simulink model "ntm"  (R2020a)
settings: Solver=VariableStepAuto  StartTime=0.0  StopTime=300  RelTol=1e-3
undefined symbols (not defined in the file or in its folder): National_Instruments, PCI
libraries: sldrtlib x5, simulink x2
settings Model: Creator=m_olivei  LastModifiedBy=m_olivei

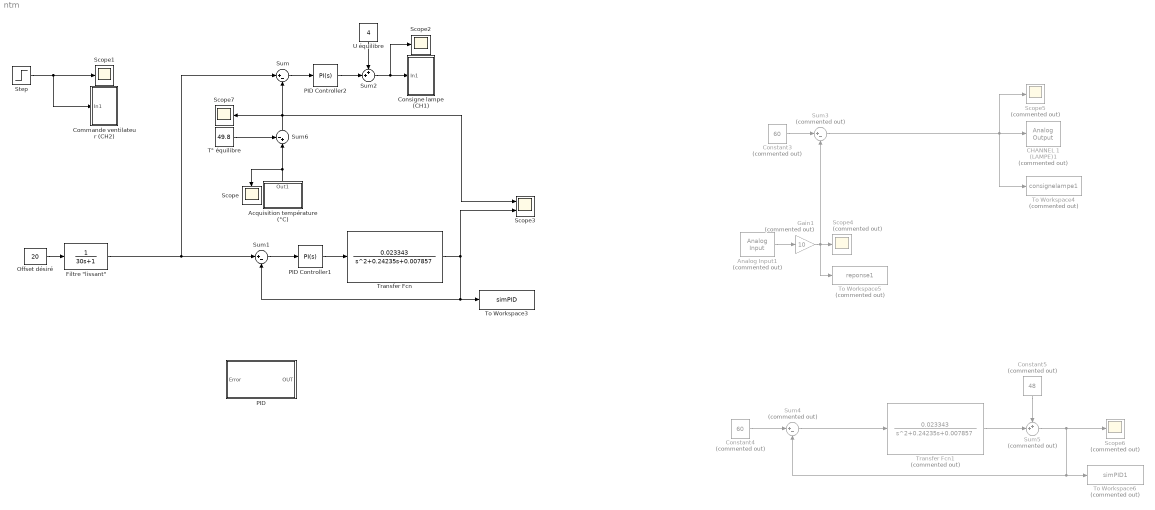
== system ntm ==
  Acquisition température (°C) : Subsystem
  Analog Input1 : sldrtlib/Analog Input  Commented=on  SampleTime=0.1  MaxMissedTicks=10  ShowMissedTicks=off  YieldWhenWaiting=off  DrvName=National_Instruments/PCI-6024E  DrvAddress=4294967295  DrvOptions=[0 0 0 0 0 0]  Channels=1  RangeMode=1  VoltRange=1  DataType=1
      settings: AttributesFormatString=National Instruments\nPCI-6024E [auto]
  CHANNEL 1 (LAMPE)1 : sldrtlib/Analog Output  Commented=on  SampleTime=0.1  MaxMissedTicks=10  ShowMissedTicks=off  YieldWhenWaiting=off  DrvName=National_Instruments/PCI-6024E  DrvAddress=4294967295  DrvOptions=[0 0 0 0 0 0]  Channels=1  RangeMode=1  VoltRange=1  InitialValue=[]  FinalValue=4
      settings: AttributesFormatString=National Instruments\nPCI-6024E [auto]
  Commande ventilateur (CH2) : Subsystem
  Consigne lampe (CH1) : Subsystem
  Constant3 : Constant  Commented=on  Value=60
  Constant4 : Constant  Commented=on  Value=60
  Constant5 : Constant  Commented=on  Value=48
  "Filtre \"lissant\"" : TransferFcn  Denominator=[30 1]
  Gain1 : Gain  Commented=on  Gain=10
  Offset désiré : Constant  Value=20
  PID : Subsystem
  PID Controller1 : simulink/Continuous/PID Controller  Controller=PI  Form=Parallel  TimeDomain=Continuous-time  UseExternalTs=off  SampleTime=-1  IntegratorMethod=Forward Euler  FilterMethod=Forward Euler  ControllerParametersSource=internal  P=0.134524809636123  I=0.0118548404136242  D=0  UseFilter=on  N=100  TunerSelectOption=Transfer Function Based (PID Tuner App)  InitialConditionSource=internal  InitialConditionForIntegrator=0  InitialConditionForFilter=0  DifferentiatorICPrevScaledInput=0  ExternalReset=none  TrackingMode=off  Kt=1  LimitOutput=on  UpperSaturationLimit=10  LowerSaturationLimit=0  LinearizeAsGain=on  AntiWindupMode=back-calculation  Kb=0.0118548404136242  POutMin=[]  POutMax=[]  IOutMin=[]  IOutMax=[]  DOutMin=[]  DOutMax=[]  NOutMin=[]  NOutMax=[]  SumOutMin=[]  SumOutMax=[]  SaturationOutMin=[]  SaturationOutMax=[]  PParamMin=[]  PParamMax=[]  IParamMin=[]  IParamMax=[]  DParamMin=[]  DParamMax=[]  NParamMin=[]  NParamMax=[]  KbParamMin=[]  KbParamMax=[]  KtParamMin=[]  KtParamMax=[]  KbOutMin=[]  KbOutMax=[]  KtOutMin=[]  KtOutMax=[]  IntegratorOutMin=[]  IntegratorOutMax=[]  FilterOutMin=[]  FilterOutMax=[]  SumI1OutMin=[]  SumI1OutMax=[]  SumI2OutMin=[]  SumI2OutMax=[]  SumI3OutMin=[]  SumI3OutMax=[]  SumI4OutMin=[]  SumI4OutMax=[]  SumDOutMin=[]  SumDOutMax=[]  DifferentiatorOutMin=[]  DifferentiatorOutMax=[]  FilterDiffOutCoefMin=[]  FilterDiffOutCoefMax=[]  ReciprocalOutMin=[]  ReciprocalOutMax=[]  SumDenOutMin=[]  SumDenOutMax=[]  SumNumOutMin=[]  SumNumOutMax=[]  DivideOutMin=[]  DivideOutMax=[]  UdiffTsProdOutMin=[]  UdiffTsProdOutMax=[]  NTsProdOutMin=[]  NTsProdOutMax=[]  UintegralTsProdOutMin=[]  UintegralTsProdOutMax=[]  UngainTsProdOutMin=[]  UngainTsProdOutMax=[]  IntegratorContinuousStateAttributes=''  IntegratorStateMustResolveToSignalObject=off  IntegratorRTWStateStorageClass=Auto  FilterContinuousStateAttributes=''  FilterStateMustResolveToSignalObject=off  FilterRTWStateStorageClass=Auto  ParallelPVariant=InternalParameters  IdealPVariant=Disabled  IVariant=InternalParameters  DVariant=Disabled  IntegratorVariant=Continuous  SatVariant=Enabled  AWVariant=BackCalculation  PCopyVariant=Disabled  TRVariant=Disabled  FdbkBlocksVariant=Forward  IdealPFdbkVariant=Disabled  SatFdbkVariant=Disabled  DerivativeFilterVariant=Disabled  NVariant=Disabled  NCopyVariant=Disabled_SignalSpec  FilterICVariant=Disabled  IntegratorICVariant=InternalICs  ExternalResetVariant=Disabled  TRSumVariant=Passthrough  SumFdbkVariant=Disabled  SumVariant=Sum_PI  TsampFilterVariant=InternalTs  TsampNgainVariant=Passthrough  TsampIntegralVariant=Passthrough
  PID Controller2 : simulink/Continuous/PID Controller  Controller=PI  Form=Parallel  TimeDomain=Continuous-time  UseExternalTs=off  SampleTime=-1  IntegratorMethod=Forward Euler  FilterMethod=Forward Euler  ControllerParametersSource=internal  P=0.134524809636123  I=0.0118548404136242  D=0  UseFilter=on  N=100  TunerSelectOption=Transfer Function Based (PID Tuner App)  InitialConditionSource=internal  InitialConditionForIntegrator=0  InitialConditionForFilter=0  DifferentiatorICPrevScaledInput=0  ExternalReset=none  TrackingMode=off  Kt=1  LimitOutput=on  UpperSaturationLimit=6  LowerSaturationLimit=0  LinearizeAsGain=on  AntiWindupMode=back-calculation  Kb=0.0118548404136242  POutMin=[]  POutMax=[]  IOutMin=[]  IOutMax=[]  DOutMin=[]  DOutMax=[]  NOutMin=[]  NOutMax=[]  SumOutMin=[]  SumOutMax=[]  SaturationOutMin=[]  SaturationOutMax=[]  PParamMin=[]  PParamMax=[]  IParamMin=[]  IParamMax=[]  DParamMin=[]  DParamMax=[]  NParamMin=[]  NParamMax=[]  KbParamMin=[]  KbParamMax=[]  KtParamMin=[]  KtParamMax=[]  KbOutMin=[]  KbOutMax=[]  KtOutMin=[]  KtOutMax=[]  IntegratorOutMin=[]  IntegratorOutMax=[]  FilterOutMin=[]  FilterOutMax=[]  SumI1OutMin=[]  SumI1OutMax=[]  SumI2OutMin=[]  SumI2OutMax=[]  SumI3OutMin=[]  SumI3OutMax=[]  SumI4OutMin=[]  SumI4OutMax=[]  SumDOutMin=[]  SumDOutMax=[]  DifferentiatorOutMin=[]  DifferentiatorOutMax=[]  FilterDiffOutCoefMin=[]  FilterDiffOutCoefMax=[]  ReciprocalOutMin=[]  ReciprocalOutMax=[]  SumDenOutMin=[]  SumDenOutMax=[]  SumNumOutMin=[]  SumNumOutMax=[]  DivideOutMin=[]  DivideOutMax=[]  UdiffTsProdOutMin=[]  UdiffTsProdOutMax=[]  NTsProdOutMin=[]  NTsProdOutMax=[]  UintegralTsProdOutMin=[]  UintegralTsProdOutMax=[]  UngainTsProdOutMin=[]  UngainTsProdOutMax=[]  IntegratorContinuousStateAttributes=''  IntegratorStateMustResolveToSignalObject=off  IntegratorRTWStateStorageClass=Auto  FilterContinuousStateAttributes=''  FilterStateMustResolveToSignalObject=off  FilterRTWStateStorageClass=Auto  ParallelPVariant=InternalParameters  IdealPVariant=Disabled  IVariant=InternalParameters  DVariant=Disabled  IntegratorVariant=Continuous  SatVariant=Enabled  AWVariant=BackCalculation  PCopyVariant=Disabled  TRVariant=Disabled  FdbkBlocksVariant=Forward  IdealPFdbkVariant=Disabled  SatFdbkVariant=Disabled  DerivativeFilterVariant=Disabled  NVariant=Disabled  NCopyVariant=Disabled_SignalSpec  FilterICVariant=Disabled  IntegratorICVariant=InternalICs  ExternalResetVariant=Disabled  TRSumVariant=Passthrough  SumFdbkVariant=Disabled  SumVariant=Sum_PI  TsampFilterVariant=InternalTs  TsampNgainVariant=Passthrough  TsampIntegralVariant=Passthrough
  Scope{,1..2,7} (4 alike) : Scope
  Scope3 : Scope  NumInputPorts=2
  Scope4 : Scope  Commented=on
  Scope5 : Scope  Commented=on
  Scope6 : Scope  Commented=on
  Step : Step  SampleTime=0
  Sum : Sum  Inputs=|+-
  Sum1 : Sum  Inputs=|+-
  Sum2 : Sum  Inputs=++|
  Sum3 : Sum  Commented=on  Inputs=|+-
  Sum4 : Sum  Commented=on  Inputs=|+-
  Sum5 : Sum  Commented=on  Inputs=++|
  Sum6 : Sum  Inputs=-+|
  To Workspace3 : ToWorkspace  VariableName=simPID  SaveFormat=Timeseries  SampleTime=-1
  To Workspace4 : ToWorkspace  Commented=on  VariableName=consignelampe1  SaveFormat=Timeseries  SampleTime=-1
  To Workspace5 : ToWorkspace  Commented=on  VariableName=reponse1  SaveFormat=Timeseries  SampleTime=-1
  To Workspace6 : ToWorkspace  Commented=on  VariableName=simPID1  SaveFormat=Timeseries  SampleTime=-1
  Transfer Fcn : TransferFcn  Numerator=[0.023343]  Denominator=[1 0.24235 0.007857]
  Transfer Fcn1 : TransferFcn  Commented=on  Numerator=[0.023343]  Denominator=[1 0.24235 0.007857]
  T° équilibre : Constant  Value=49.8
  U équilibre : Constant  Value=4
  wires:
  Step/1 -> Commande ventilateur (CH2)/1(In1), Scope1/1
  Sum1/1 -> PID Controller1/1
  Offset désiré/1 -> "Filtre \"lissant\""/1
  PID Controller2/1 -> Sum2/2
  Sum3/1 -> To Workspace4/1, Scope5/1, CHANNEL 1 (LAMPE)1/1
  Gain1/1 -> Sum3/2, To Workspace5/1, Scope4/1
  Analog Input1/1 -> Gain1/1
  Constant3/1 -> Sum3/1
  Sum4/1 -> Transfer Fcn1/1
  Sum5/1 -> Scope6/1, To Workspace6/1, Sum4/2
  Constant5/1 -> Sum5/1
  Transfer Fcn1/1 -> Sum5/2
  Constant4/1 -> Sum4/1
  Sum/1 -> PID Controller2/1
  U équilibre/1 -> Sum2/1
  Sum2/1 -> Consigne lampe (CH1)/1(In1), Scope2/1
  Sum6/1 -> Scope3/1, Sum/2, Scope7/1
  T° équilibre/1 -> Sum6/1
  Transfer Fcn/1 -> Scope3/2, Sum1/2, To Workspace3/1
  PID Controller1/1 -> Transfer Fcn/1
  "Filtre \"lissant\""/1 -> Sum/1, Sum1/1
  Acquisition température (°C)/1(Out1) -> Sum6/2, Scope/1

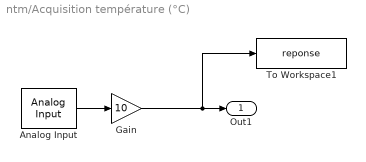
== system ntm/Acquisition température (°C) ==
  Analog Input : sldrtlib/Analog Input  SampleTime=0.1  MaxMissedTicks=10  ShowMissedTicks=off  YieldWhenWaiting=off  DrvName=National_Instruments/PCI-6024E  DrvAddress=4294967295  DrvOptions=[0 0 0 0 0 0]  Channels=1  RangeMode=1  VoltRange=1  DataType=1
      settings: AttributesFormatString=National Instruments\nPCI-6024E [auto]
  Gain : Gain  Gain=10
  To Workspace1 : ToWorkspace  VariableName=reponse  SaveFormat=Timeseries  SampleTime=-1
  Out1 : Outport
  wires:
  Analog Input/1 -> Gain/1
  Gain/1 -> To Workspace1/1, Out1/1

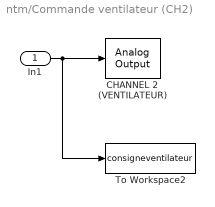
== system ntm/Commande ventilateur (CH2) ==
  In1 : Inport
  CHANNEL 2 (VENTILATEUR) : sldrtlib/Analog Output  SampleTime=0.1  MaxMissedTicks=10  ShowMissedTicks=off  YieldWhenWaiting=off  DrvName=National_Instruments/PCI-6024E  DrvAddress=4294967295  DrvOptions=[0 0 0 0 0 0]  Channels=2  RangeMode=1  VoltRange=1  InitialValue=[]  FinalValue=1
      settings: AttributesFormatString=National Instruments\nPCI-6024E [auto]
  To Workspace2 : ToWorkspace  VariableName=consigneventilateur  SaveFormat=Timeseries  SampleTime=-1
  wires:
  In1/1 -> To Workspace2/1, CHANNEL 2 (VENTILATEUR)/1

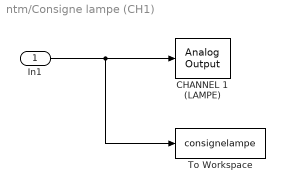
== system ntm/Consigne lampe (CH1) ==
  In1 : Inport
  CHANNEL 1 (LAMPE) : sldrtlib/Analog Output  SampleTime=0.1  MaxMissedTicks=10  ShowMissedTicks=off  YieldWhenWaiting=off  DrvName=National_Instruments/PCI-6024E  DrvAddress=4294967295  DrvOptions=[0 0 0 0 0 0]  Channels=1  RangeMode=1  VoltRange=1  InitialValue=[]  FinalValue=4
      settings: AttributesFormatString=National Instruments\nPCI-6024E [auto]
  To Workspace : ToWorkspace  VariableName=consignelampe  SaveFormat=Timeseries  SampleTime=-1
  wires:
  In1/1 -> To Workspace/1, CHANNEL 1 (LAMPE)/1

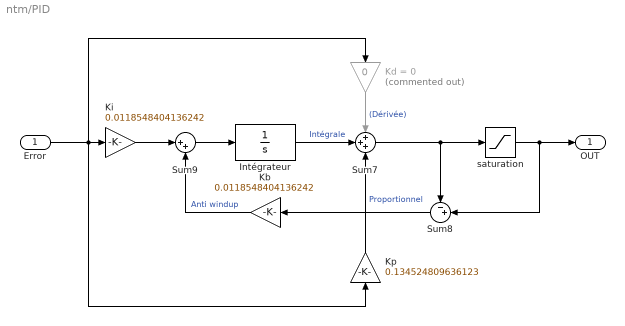
== system ntm/PID ==
  Error : Inport
  Intégrateur : TransferFcn  Denominator=[1 0]
  Kb : Gain  Gain=0.0118548404136242
  Kd = 0 : Gain  Commented=on  Gain=0
  Ki : Gain  Gain=0.0118548404136242
  Kp : Gain  Gain=0.134524809636123
  Sum7 : Sum  Inputs=+++
  Sum8 : Sum  Inputs=-+|
  Sum9 : Sum  Inputs=|++
  saturation : Saturate  UpperLimit=6  LowerLimit=0
  OUT : Outport
  wires:
  Kd = 0/1 -> Sum7/1  "(Dérivée)"
  Kp/1 -> Sum7/3  "Proportionnel"
  Sum7/1 -> Sum8/1, saturation/1
  Sum9/1 -> Intégrateur/1
  Kb/1 -> Sum9/2  "Anti windup"
  saturation/1 -> OUT/1, Sum8/2
  Sum8/1 -> Kb/1
  Ki/1 -> Sum9/1
  Intégrateur/1 -> Sum7/2  "Intégrale"
  Error/1 -> Kd = 0/1, Kp/1, Ki/1
